simulink model "simulation_upgrade"  (R2024b)
settings: Solver=ode1be  StartTime=0.0  StopTime=10  FixedStep=0.001  RelTol=1e-3
model workspace (MAT data in the model file):
  AMP = 1
  FREQ = 1
  i_abc = 1
values from neighbouring files (symbols this model uses):
  v_WLTP = [0 0 0 0 0 0 0 0 0 0 0 0 ... (180001 elements, 1x180001)]    [v_WLTP.mat]
undefined symbols (not defined in the file or in its folder): A, a_sig, b_sig, C1, C2, C3, Cd, CG_z, downshift, Drive_wheel, Driveshaft, f_blend, f_OVD, fo, front_seat_dist, fs, g, Gearbox, i, i_sig, Inclination, Inertia, Jr2, K, m, M_curve_1, M_curve_2, m_driver, M_N_1, M_N_2, mi_c, mi_s, Mode, N_clutch, n_curve_1, n_curve_2, n_driver, n_max_1, n_max_2, n_shift, n_surfaces, Pl, Planetary, r_eq_clutch, r_geom, r_wheel, rho, Shaft, shift_time, sigma0, sigma1, sigma2, slope_angle, Stage1, Stage2, Stage3, upshift, v0, vel_wind, vs ... (+5)
libraries: simulink x29, slpidlib x3
(part 6 of 9)

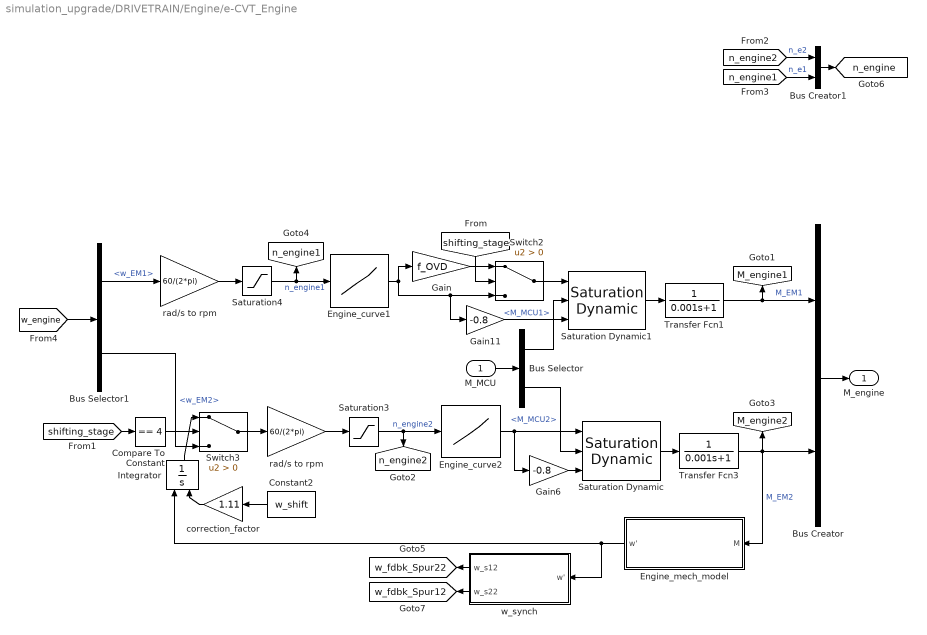
== system simulation_upgrade/DRIVETRAIN/Engine/e-CVT_Engine ==
  M_MCU : Inport
  Bus Creator : BusCreator  Inputs=2
  Bus Creator1 : BusCreator  Inputs=2
  Bus Selector : BusSelector  OutputSignals=M_MCU1,M_MCU2
  Bus Selector1 : BusSelector  OutputSignals=w_EM1,w_EM2
  Compare To Constant : simulink/Logic and Bit Operations/Compare To Constant  relop===  const=4  OutDataTypeStr=boolean
  Constant2 : Constant  Value=w_shift
  Engine_curve1 : Lookup_n-D  NumberOfTableDimensions=1  BreakpointsForDimension1=n_curve_1  Table=M_curve_1  InternalRulePriority=Speed  RndMeth=Simplest
  Engine_curve2 : Lookup_n-D  NumberOfTableDimensions=1  BreakpointsForDimension1=n_curve_2  Table=M_curve_2  InternalRulePriority=Speed  RndMeth=Simplest
  Engine_mech_model : Subsystem  mask{J_S1=Stage1.Spur1.J, J_S2=Stage1.Spur2.J, J_S11=Stage2.Spur11.J, J_S21=Stage2.Spur21.J, J_S12=Stage2.Spur12.J, J_S22=Stage2.Spur22.J, Jshaft=Shaft.J}
      mask prompts: J_S1 "Stage 1 Spur 1 Inertia"; J_S2 "Stage 1 Spur 2 Inertia"; J_S11 "Stage 2 Spur 11 Inertia"; J_S21 "Stage 2 Spur 21 Inertia"; J_S12 "Stage 2 Spur 12 Inertia"; J_S22 "Stage 2 Spur 22 Inertia"; Jshaft "Shaft Inertia"
  Gain : Gain  Gain=f_OVD
  Gain11 : Gain  Gain=-0.8
  Gain6 : Gain  Gain=-0.8
  Integrator : Integrator  InitialConditionSource=external
  Saturation Dynamic : simulink/Discontinuities/Saturation Dynamic  OutMin=[]  OutMax=[]  OutDataTypeStr=Inherit: Same as second input  OutDataType=fixdt(1, 16)  OutScaling=2^-10  DoSatur=off
  Saturation Dynamic1 : simulink/Discontinuities/Saturation Dynamic  OutMin=[]  OutMax=[]  OutDataTypeStr=Inherit: Same as second input  OutDataType=fixdt(1, 16)  OutScaling=2^-10  DoSatur=off
  Saturation3 : Saturate  UpperLimit=n_max_2
  Saturation4 : Saturate  UpperLimit=n_max_2
  Switch2 : Switch  Criteria=u2 > Threshold  SaturateOnIntegerOverflow=off  InputSameDT=off
  Switch3 : Switch  Criteria=u2 > Threshold  SaturateOnIntegerOverflow=off  InputSameDT=off
  Transfer Fcn1 : TransferFcn  Denominator=[0.001 1]
  Transfer Fcn3 : TransferFcn  Denominator=[0.001 1]
  "correction_factor " : Gain  Gain=1.11
  rad/s to rpm : Gain  Gain=60/(2*pi)
  "rad/s to rpm " : Gain  Gain=60/(2*pi)
  w_synch : Subsystem
      settings: PortSchema="{\"entries\":[{\"content\":{\"sides\":[{\"content\":{\"connectorIds\":[\"Out1\",\"Out2\"]},\"type\":\"ConnectorPlacement.EquallySpacedRectSide\",\"uuid\":\"0c74f9d6-4dd7-46ca-984a-3872ca362183\"},{\"content\":{\"connectorIds\":[\"In1\"],\"side\":\"RIGHT\"},\"type\":\"ConnectorPlacement.EquallySpacedRectSide\",\"uuid\":\"545eaab0-161e-407a-bd7a-8511cf00bcf5\"},{\"content\":{\"side\":\"TOP\"},\"type\":\"ConnectorPlacement.EquallySpacedRectSide\",\"uuid\":\"a44ef98a-c6fa-4a8f-9ec6-3c467f201227\"}]},\"type\":\"ConnectorPlacement.EquallySpacedConnector\",\"uuid\":\"6cdff010-dc2a-4ca6-852d-068deaf42780\"}],\"packageUris\":[\"http://schema.mathworks.com/mf0/Connector/R2020b\"],\"version\":\"1.0\"}"
      mask Display: image('branco.png');
  M_engine : Outport
  tag scope: M_engine1=global, M_engine2=global, n_engine1=global, n_engine2=global, n_engine=global, w_fdbk_Spur12=global, w_fdbk_Spur22=global
  wires:
  w_synch/2(w_s22) -> [w_fdbk_Spur12]
  w_synch/1(w_s12) -> [w_fdbk_Spur22]
  Gain11/1 -> Saturation Dynamic1/3
  rad/s to rpm/1 -> Saturation4/1
  Saturation4/1 -> [n_engine1], Engine_curve1/1  "n_engine1"
  Saturation Dynamic1/1 -> Transfer Fcn1/1
  "correction_factor "/1 -> Integrator/2
  Constant2/1 -> "correction_factor "/1
  Bus Selector1/2 -> Switch3/3  "<w_EM2>"
  Saturation Dynamic/1 -> Transfer Fcn3/1
  Gain6/1 -> Saturation Dynamic/3
  Bus Creator1/1 -> [n_engine]
  [n_engine1] -> Bus Creator1/2  "n_e1"
  [n_engine2] -> Bus Creator1/1  "n_e2"
  Integrator/1 -> Switch3/1
  Transfer Fcn3/1 -> [M_engine2], Engine_mech_model/1(M), Bus Creator/2  "M_EM2"
  Engine_mech_model/1(w') -> Integrator/1, w_synch/1(w')
  [shifting_stage] -> Compare To Constant/1
  Compare To Constant/1 -> Switch3/2
  Switch3/1 -> "rad/s to rpm "/1
  [shifting_stage] -> Switch2/2
  Gain/1 -> Switch2/1
  Switch2/1 -> Saturation Dynamic1/1
  Bus Creator/1 -> M_engine/1
  [w_engine] -> Bus Selector1/1
  Bus Selector/2 -> Saturation Dynamic/2  "<M_MCU2>"
  Saturation3/1 -> [n_engine2], Engine_curve2/1  "n_engine2"
  Engine_curve2/1 -> Saturation Dynamic/1, Gain6/1
  "rad/s to rpm "/1 -> Saturation3/1
  Bus Selector1/1 -> rad/s to rpm/1  "<w_EM1>"
  M_MCU/1 -> Bus Selector/1
  Bus Selector/1 -> Saturation Dynamic1/2  "<M_MCU1>"
  Engine_curve1/1 -> Gain/1, Gain11/1, Switch2/3
  Transfer Fcn1/1 -> [M_engine1], Bus Creator/1  "M_EM1"

== system simulation_upgrade/DRIVETRAIN/Transmission/Differential and Driveshafts ==
  M_Diff : Inport
  Bus Creator : BusCreator  Inputs=4
  Gain2 : Gain  Gain=0.5
  Gain3 : Gain  Gain=0.5
  Gain4 : Gain  Gain=0.5
  Sum : Sum  Inputs=+|+
  Torsional_stiffness_left_output_shaft : Subsystem  mask{c=Driveshaft.Right.c, d=Driveshaft.Right.d, J=Driveshaft.Right.J}
      mask prompts: c "Shaft_Stiffness_Nm/rad"; d "Shaft_Damping_Nms/rad"; J "Inertia_kgm^2"
      settings: PortSchema="{\"entries\":[{\"content\":{\"sides\":[{\"content\":{\"connectorIds\":[\"In1\",\"Out2\"]},\"type\":\"ConnectorPlacement.EquallySpacedRectSide\",\"uuid\":\"898fedf9-82f7-4bc2-bf05-880de36b191d\"},{\"content\":{\"connectorIds\":[\"Out1\",\"In2\"],\"side\":\"RIGHT\"},\"type\":\"ConnectorPlacement.EquallySpacedRectSide\",\"uuid\":\"50317b6c-245f-4bd1-a8cd-7a774957ae86\"},{\"content\":{\"side\":\"TOP\"},\"type\":\"ConnectorPlacement.EquallySpacedRectSide\",\"uuid\":\"ff1de2a1-7305-40d8-9e1f-fd0fa1e7d830\"}]},\"type\":\"ConnectorPlacement.EquallySpacedConnector\",\"uuid\":\"6ce82d73-f3da-4f59-9039-464a6ef3e9c5\"}],\"packageUris\":[\"http://schema.mathworks.com/mf0/Connector/R2020b\"],\"version\":\"1.0\"}"
      mask Display: image('images/torsion.png');
  Torsional_stiffness_right_output_shaft : Subsystem  mask{c=Driveshaft.Right.c, d=Driveshaft.Right.d, J=Driveshaft.Right.J}
      mask prompts: c "Shaft_Stiffness_Nm/rad"; d "Shaft_Damping_Nms/rad"; J "Inertia_kgm^2"
      settings: PortSchema="{\"entries\":[{\"content\":{\"sides\":[{\"content\":{\"connectorIds\":[\"In1\",\"Out2\"]},\"type\":\"ConnectorPlacement.EquallySpacedRectSide\",\"uuid\":\"898fedf9-82f7-4bc2-bf05-880de36b191d\"},{\"content\":{\"connectorIds\":[\"Out1\",\"In2\"],\"side\":\"RIGHT\"},\"type\":\"ConnectorPlacement.EquallySpacedRectSide\",\"uuid\":\"50317b6c-245f-4bd1-a8cd-7a774957ae86\"},{\"content\":{\"side\":\"TOP\"},\"type\":\"ConnectorPlacement.EquallySpacedRectSide\",\"uuid\":\"ff1de2a1-7305-40d8-9e1f-fd0fa1e7d830\"}]},\"type\":\"ConnectorPlacement.EquallySpacedConnector\",\"uuid\":\"6ce82d73-f3da-4f59-9039-464a6ef3e9c5\"}],\"packageUris\":[\"http://schema.mathworks.com/mf0/Connector/R2020b\"],\"version\":\"1.0\"}"
      mask Display: image('images/torsion.png');
  eff : Gain  Gain=0.98
  "eff " : Gain  Gain=0.98
  M_tra : Outport
  tag scope: M_diff=global, M_tra=global, w_fdbk_axleL=global, w_fdbk_axleR=global, w_fdbk_diff=global
  wires:
  "eff "/1 -> Bus Creator/4  "M_axleR"
  eff/1 -> Bus Creator/1  "M_axleL"
  Bus Creator/1 -> M_tra/1, [M_tra]
  [M_diff] -> Bus Creator/3
  [M_GB] -> Bus Creator/2
  [w_fdbk_tire] -> Torsional_stiffness_left_output_shaft/2(Speed_fdbk), Torsional_stiffness_right_output_shaft/2(Speed_fdbk)
  Torsional_stiffness_right_output_shaft/1(Torque_out) -> "eff "/1
  Torsional_stiffness_left_output_shaft/1(Torque_out) -> eff/1
  Sum/1 -> Gain3/1
  Gain4/1 -> Torsional_stiffness_right_output_shaft/1(Torque_in)  "M_axleR"
  Torsional_stiffness_left_output_shaft/2(phi_shaft_R_dot) -> Sum/1, [w_fdbk_axleL]
  Gain3/1 -> [w_fdbk_diff]
  M_Diff/1 -> Gain4/1, Gain2/1, [M_diff]  "M_diff"
  Torsional_stiffness_right_output_shaft/2(phi_shaft_R_dot) -> [w_fdbk_axleR], Sum/2
  Gain2/1 -> Torsional_stiffness_left_output_shaft/1(Torque_in)  "M_axleL"

== system simulation_upgrade/DRIVETRAIN/Transmission/Gearbox ==
  note: 1) Add Subsystem or Model blocks as valid variant choices.
      | 2) You cannot connect blocks at this level. At simulation, connectivity is automatically
      | determined, based on the active variant and port name matching.
  M_engine : Inport
  AMT : Subsystem  VariantControl=Gearbox == 2
      mask Display: image('images/clutch.jpg');
  AT : Subsystem  VariantControl=Gearbox == 1
      mask Display: image('images/planetary.png');
  DCT : Subsystem  VariantControl=Gearbox == 3
      mask Display: image('images/dual_clutch.png');
  TDT : Subsystem  VariantControl=Gearbox == 4
      mask Display: image('images/dog_clutch.png');
  e-CVT : Subsystem  VariantControl=Gearbox == 5
      mask Display: image('images/e-CVT.png');
  M_Diff : Outport

== system simulation_upgrade/DRIVETRAIN/Wheel Model/Front Wheels ==
  Vload : Inport
  M_tra : Inport  Port=2
  M_break : Inport  Port=3
  Divide1 : Product  Inputs=/*
  Dynamic Radius : Subsystem
  Wheel Torque : Subsystem
  F_front_wheels : Outport
  wires:
  M_tra/1 -> Wheel Torque/1(M_tra)
  M_break/1 -> Wheel Torque/2(M_break)
  Wheel Torque/1(M_front_wheels) -> Divide1/2
  Vload/1 -> Dynamic Radius/1(V_load)
  Dynamic Radius/1(r_dynamic_front) -> Divide1/1
  Divide1/1 -> F_front_wheels/1

== system simulation_upgrade/DRIVETRAIN/Wheel Model/Rear Wheels ==
  M_tra : Inport
  M_break : Inport  Port=2
  Vload : Inport  Port=3
  Divide1 : Product  Inputs=/*
  Dynamic Radius : Subsystem
  Wheel Torque : Subsystem
  F_rear_wheels : Outport
  wires:
  Vload/1 -> Dynamic Radius/1(V_load)
  Divide1/1 -> F_rear_wheels/1
  Dynamic Radius/1(r_dynamic_rear) -> Divide1/1
  M_tra/1 -> Wheel Torque/1(M_tra)
  M_break/1 -> Wheel Torque/2(M_break)
  Wheel Torque/1(M_rear_wheels) -> Divide1/2

== system simulation_upgrade/DYNAMICS/Vehicle Dynamics/Effective mass ==
  " 2nd engine gearbox inertia" : Constant  Commented=on  Value=Inertia.Second_Engine_Gearbox
  Add : Sum
  Add1 : Sum  Commented=on  Inputs=+++
  Add2 : Sum  Commented=on
  Add3 : Sum  Commented=on  Inputs=+++
  Add4 : Sum  Commented=on
  Add5 : Sum  Commented=on
  Constant : Constant  Value=m
  Constant1 : Constant  Commented=on  Value=r_wheel
  Divide : Product  Commented=on  Inputs=*/
  From : From  Commented=on  GotoTag=C2_ist  TagVisibility=global
  Manual Switch : ManualSwitch
  Multiport Switch : MultiPortSwitch  Commented=on  DataPortOrder=Zero-based contiguous  zeroidx=on  SaturateOnIntegerOverflow=off  InputSameDT=off
  Output shaft inertia : Constant  Commented=on  Value=Inertia.Output_Shaft
  Scope : Scope
  Square : Math  Commented=on  Operator=square
  Stage 1 - 1st Gear Inertia : Constant  Commented=on  Value=Inertia.Gearbox1.Stage_1_1st_Gear
  Stage 1 - 2nd Gear Inertia1 : Constant  Commented=on  Value=Inertia.Gearbox1.Stage_1_2nd_Gear
  Stage 2 - 1st Gear Inertia : Constant  Commented=on  Value=Inertia.Gearbox1.Stage_2_1st_Gear
  Stage 2 - 2nd Gear Inertia : Constant  Commented=on  Value=Inertia.Gearbox1_Stage_2_2nd_Gear
  Stage 3 : Constant  Commented=on  Value=Inertia.Gearbox1_Stage_3
  m_eff : Outport
  tag scope: m_eff=global
  wires:
  Add/1 -> Manual Switch/2
  Add4/1 -> Multiport Switch/3  "1st gear"
  Multiport Switch/1 -> Divide/1  "I_eff"
  Divide/1 -> Add/2
  Square/1 -> Divide/2
  Add5/1 -> Multiport Switch/4  "2nd gear"
  Output shaft inertia/1 -> Add2/1
  From/1 -> Multiport Switch/1
  Add2/1 -> Add5/1, Add4/1, Multiport Switch/2  "neutral"
  Constant/1 -> Manual Switch/1, Add/1
  Constant1/1 -> Square/1
  Add3/1 -> Add5/2  "2nd gear gearbox inertia"
  Add1/1 -> Add4/2  "1st gear gearbox inertia"
  " 2nd engine gearbox inertia"/1 -> Add2/2
  Stage 1 - 1st Gear Inertia/1 -> Add1/1
  Stage 3/1 -> Add1/3, Add3/1
  Stage 2 - 1st Gear Inertia/1 -> Add1/2
  Stage 2 - 2nd Gear Inertia/1 -> Add3/3
  Stage 1 - 2nd Gear Inertia1/1 -> Add3/2
  Manual Switch/1 -> Scope/1, [m_eff], m_eff/1

== system simulation_upgrade/PANEL/Pretty shot/Aerodynamic Forces  ==
  " " : Inport
  "  " : Outport
  wires:
  " "/1 -> "  "/1

== system simulation_upgrade/PANEL/Pretty shot/Engine(s)  ==
  "  " : Inport
  "             " : Outport
  "              " : Outport  Port=2
  wires:
  "  "/1 -> "             "/1

== system simulation_upgrade/PANEL/Pretty shot/Inclination  ==
  Constant : Constant
  "   " : Outport
  " " : Outport  Port=2
  wires:
  Constant/1 -> " "/1, "   "/1

== system simulation_upgrade/PANEL/Pretty shot/Load Transfer  ==
  " " : Inport
  "      " : Inport  Port=2
  Terminator : Terminator
  "  " : Outport
  wires:
  "      "/1 -> Terminator/1
  " "/1 -> "  "/1

== system simulation_upgrade/PANEL/Pretty shot/Main Control Unit  ==
  " " : Inport
  "   " : Inport  Port=2
  Chart : Stateflow chart  Commented=on  TreatAsAtomicUnit=on
  "  " : Outport
  "    " : Outport  Port=2
  wires:
  Chart/1("  ") -> "  "/1
  Chart/2("    ") -> "    "/1
  "   "/1 -> Chart/2("   ")
  " "/1 -> Chart/1(" ")

== system simulation_upgrade/PANEL/Pretty shot/Speed Profile  ==
  Constant : Constant
  " " : Outport
  wires:
  Constant/1 -> " "/1

== system simulation_upgrade/PANEL/Pretty shot/Speed control  ==
  "    " : Inport
  " " : Inport  Port=2
  "         " : Outport
  "        " : Outport  Port=2
  wires:
  " "/1 -> "         "/1
  "    "/1 -> "        "/1

== system simulation_upgrade/PANEL/Pretty shot/Transmission  ==
  " " : Inport
  "     " : Inport  Port=2
  "    " : Inport  Port=3
  "   " : Inport  Port=4
  Variant Subsystem : Subsystem  Commented=on  Variant=on
  "  " : Outport
  wires:
  " "/1 -> "  "/1

== system simulation_upgrade/PANEL/Pretty shot/Vehicle Dynamics  ==
  " " : Inport
  "  " : Outport
  wires:
  " "/1 -> "  "/1

== system simulation_upgrade/PANEL/Pretty shot/Wheel Model  ==
  "  " : Inport
  " " : Inport  Port=2
  "   " : Outport
  "    " : Outport  Port=2
  wires:
  "  "/1 -> "    "/1
  " "/1 -> "   "/1

== system simulation_upgrade/CONTROLS/Main Control Unit/AMT_MCU/Subsystem ==
  clutchSet : Inport
  Clock : Clock
  Delay : Delay  DelayLength=1  InitialCondition=1  InputProcessing=Columns as channels (frame based)
  Equal1 : RelationalOperator  Operator=<=  OutDataTypeStr=boolean  RndMeth=Simplest  InputSameDT=off
  Equal2 : RelationalOperator  OutDataTypeStr=boolean  RndMeth=Simplest  InputSameDT=off
  Manual Switch1 : ManualSwitch
  Polynomial : Subsystem
  Product : Product
  Scope : Scope  NumInputPorts=3
  Scope2 : Scope
  Scope3 : Scope
  Sigmoid : Subsystem
  Sum : Sum  Inputs=|-+
  Sum2 : Sum  Inputs=++|
  Switch : Switch  Criteria=u2 > Threshold  SaturateOnIntegerOverflow=off  InputSameDT=off
  Switch1 : Switch  Threshold=1  SaturateOnIntegerOverflow=off  InputSameDT=off
  Transport Delay : TransportDelay  DelayTime=0.001  InitialOutput=1
  signal_register : Subsystem
  time_register : Subsystem
  C2 : Outport
  wires:
  Sum/1 -> Sigmoid/1(" "), Polynomial/1(" ")
  Switch1/1 -> Transport Delay/1
  Product/1 -> Sum2/2
  time_register/1(t0) -> Scope2/1, Sum/1
  Equal2/1 -> Switch/3
  Clock/1 -> time_register/1(t), Sum/2
  Delay/1 -> Scope3/1, time_register/Trigger, signal_register/1(signal), signal_register/Trigger, Scope/3, Switch1/1, Equal2/1, Equal1/1
  clutchSet/1 -> Delay/1
  Polynomial/1("  ") -> Manual Switch1/1
  signal_register/1(previous_value) -> Sum2/1
  Sigmoid/1("  ") -> Manual Switch1/2
  Transport Delay/1 -> Scope/2, C2/1
  Equal1/1 -> Switch/1
  Sum2/1 -> Equal1/2, Equal2/2, Scope/1, Switch1/3
  signal_register/2(difference) -> Switch/2, Product/1
  Manual Switch1/1 -> Product/2
  Switch/1 -> Switch1/2

== system simulation_upgrade/CONTROLS/Main Control Unit/AT_MCU/Clutch_Profile ==
  clutch2set : Inport
  clutch1set : Inport  Port=2
  Manual Switch : ManualSwitch  CurrentSetting=0
  Manual Switch1 : ManualSwitch  CurrentSetting=0
  polynomial_s_response : Subsystem
  polynomial_s_response1 : Subsystem
  sigmoid_response : Subsystem
  sigmoid_response1 : Subsystem
  Out1 : Outport
  Out2 : Outport  Port=2
  wires:
  polynomial_s_response/1(Out1) -> Manual Switch/2
  sigmoid_response/1(Out1) -> Manual Switch/1
  clutch2set/1 -> polynomial_s_response1/1(clutch2set), sigmoid_response1/1(clutch2set)
  polynomial_s_response1/1(Out1) -> Manual Switch1/2
  sigmoid_response1/1(Out1) -> Manual Switch1/1
  clutch1set/1 -> sigmoid_response/1(clutch1set), polynomial_s_response/1(clutch1set)
  Manual Switch1/1 -> Out1/1  "c2"
  Manual Switch/1 -> Out2/1  "c1"

== system simulation_upgrade/CONTROLS/Main Control Unit/AT_MCU/Shifting Impulses ==
  n_engine : Inport
  shiftng_stage : Inport  Port=2
  C2 : Inport  Port=3
  AND : Logic  Inputs=3  IconShape=distinctive  AllPortsSameDT=off  OutDataTypeStr=boolean
  AND1 : Logic  Inputs=4  IconShape=distinctive  AllPortsSameDT=off  OutDataTypeStr=boolean
  Compare To Constant : simulink/Logic and Bit Operations/Compare To Constant  relop===  const=0  OutDataTypeStr=boolean
  Compare To Constant1 : simulink/Logic and Bit Operations/Compare To Constant  relop=<  const=2000  OutDataTypeStr=boolean
  Compare To Constant2 : simulink/Logic and Bit Operations/Compare To Constant  relop=>=  const=n_shift  OutDataTypeStr=boolean
  Compare To Constant3 : simulink/Logic and Bit Operations/Compare To Constant  relop===  const=2  OutDataTypeStr=boolean
  Compare To Constant4 : simulink/Logic and Bit Operations/Compare To Constant  relop===  const=1  OutDataTypeStr=boolean
  Compare To Constant5 : simulink/Logic and Bit Operations/Compare To Constant  relop=<  const=0  OutDataTypeStr=boolean
  Delay : Delay  DelayLength=1
  Delay2 : Delay  DelayLength=1
  Manual Switch : ManualSwitch  CurrentSetting=0
  Manual Switch1 : ManualSwitch
  Scope : Scope
  Scope2 : Scope
  Zero1 : Constant  Value=0  OutDataTypeStr=Inherit: Inherit via back propagation
  downshift impulse : Subsystem
  upshift impulse : Subsystem
  upshift command : Outport
  downshift command : Outport  Port=2
  wires:
  C2/1 -> Compare To Constant3/1, Compare To Constant4/1
  Compare To Constant3/1 -> AND1/2
  AND1/1 -> downshift impulse/1(Event)
  Compare To Constant2/1 -> AND/2
  upshift impulse/1(Impulse) -> Delay2/1, Scope/1
  Compare To Constant/1 -> AND/3, AND1/1
  AND/1 -> upshift impulse/1(Event)
  downshift impulse/1(Impulse) -> Delay/1, Scope2/1
  Delay/1 -> Manual Switch/2
  Compare To Constant1/1 -> AND1/3
  Manual Switch/1 -> downshift command/1
  shiftng_stage/1 -> Compare To Constant/1
  [acc] -> Compare To Constant5/1
  n_engine/1 -> Compare To Constant1/1, Compare To Constant2/1
  Compare To Constant5/1 -> AND1/4
  Delay2/1 -> Manual Switch1/1
  Manual Switch1/1 -> upshift command/1
  Zero1/1 -> Manual Switch/1, Manual Switch1/2
  Compare To Constant4/1 -> AND/1

== system simulation_upgrade/CONTROLS/Main Control Unit/CVT_MCU/Torque Split ==
  M_Set_SC : Inport
  M_EM2 : Inport  Port=2
  GreaterThan : RelationalOperator  Operator=>  OutDataTypeStr=boolean  RndMeth=Simplest  InputSameDT=off
  M_N_2 : Step  Time=0  After=M_N_2  SampleTime=0
  Recuperation Limit : Saturate  UpperLimit=0  LowerLimit=-80
  Recuperation Limit1 : Saturate  UpperLimit=0  LowerLimit=-80
  Saturation : Saturate  UpperLimit=M_N_1  LowerLimit=0
  Saturation1 : Saturate  UpperLimit=M_N_2  LowerLimit=0
  Subtract : Sum  Inputs=+-
  Subtract1 : Sum  Inputs=-+
  Switch : Switch  Criteria=u2 > Threshold  SaturateOnIntegerOverflow=off  InputSameDT=off
  Switch2 : Switch  Criteria=u2 > Threshold  SaturateOnIntegerOverflow=off  InputSameDT=off
  M_Set_1 : Outport
  M_Set_2 : Outport  Port=2
  wires:
  Recuperation Limit1/1 -> Switch/3
  Saturation1/1 -> Switch2/1
  Subtract/1 -> Recuperation Limit1/1
  M_EM2/1 -> Subtract1/1
  Switch/1 -> M_Set_1/1
  Saturation/1 -> Switch/1
  Recuperation Limit/1 -> Subtract/2, Switch2/3
  Switch2/1 -> M_Set_2/1
  GreaterThan/1 -> Switch/2
  Subtract1/1 -> Saturation/1
  M_Set_SC/1 -> Recuperation Limit/1, Saturation1/1, Switch2/2, Subtract/1, Subtract1/2, GreaterThan/1
  M_N_2/1 -> GreaterThan/2

== system simulation_upgrade/CONTROLS/Main Control Unit/DCT_MCU/Subsystem ==
  clutchSet : Inport
  Clock : Clock
  Delay : Delay  DelayLength=1  InitialCondition=1  InputProcessing=Columns as channels (frame based)
  Equal1 : RelationalOperator  Operator=<=  OutDataTypeStr=boolean  RndMeth=Simplest  InputSameDT=off
  Equal2 : RelationalOperator  OutDataTypeStr=boolean  RndMeth=Simplest  InputSameDT=off
  Hyperbolic : Subsystem
  Manual Switch1 : ManualSwitch  CurrentSetting=0
  Polynomial : Subsystem
  Product : Product
  Scope : Scope  NumInputPorts=3
  Scope2 : Scope
  Scope3 : Scope
  Sigmoid : Subsystem
  Sum : Sum  Inputs=|-+
  Sum2 : Sum  Inputs=++|
  Switch : Switch  Criteria=u2 > Threshold  SaturateOnIntegerOverflow=off  InputSameDT=off
  Switch1 : Switch  Threshold=1  SaturateOnIntegerOverflow=off  InputSameDT=off
  Transport Delay : TransportDelay  DelayTime=0.001  InitialOutput=1
  signal_register : Subsystem
  time_register : Subsystem
  C2 : Outport
  wires:
  Sum/1 -> Hyperbolic/1(" "), Polynomial/1(" ")
  Switch1/1 -> Transport Delay/1
  Product/1 -> Sum2/2
  time_register/1(t0) -> Scope2/1, Sum/1
  Equal2/1 -> Switch/3
  Clock/1 -> time_register/1(t), Sum/2
  Polynomial/1("  ") -> Manual Switch1/1
  signal_register/1(previous_value) -> Sum2/1
  Sigmoid/1("  ") -> ?
  Transport Delay/1 -> Scope/2, C2/1
  Equal1/1 -> Switch/1
  Sum2/1 -> Equal1/2, Equal2/2, Scope/1, Switch1/3
  signal_register/2(difference) -> Switch/2, Product/1
  Manual Switch1/1 -> Product/2
  Switch/1 -> Switch1/2
  Hyperbolic/1("  ") -> Manual Switch1/2
  clutchSet/1 -> Delay/1
  Delay/1 -> time_register/Trigger, Scope/3, Switch1/1, Equal2/1, Equal1/1, signal_register/Trigger, signal_register/1(signal), Scope3/1

== system simulation_upgrade/CONTROLS/Main Control Unit/DCT_MCU/Subsystem1 ==
  clutchSet : Inport
  Clock : Clock
  Equal1 : RelationalOperator  Operator=<=  OutDataTypeStr=boolean  RndMeth=Simplest  InputSameDT=off
  Equal2 : RelationalOperator  OutDataTypeStr=boolean  RndMeth=Simplest  InputSameDT=off
  Hyperbolic : Subsystem
  Manual Switch1 : ManualSwitch
  Polynomial : Subsystem
  Product : Product
  Scope : Scope  NumInputPorts=3
  Scope2 : Scope
  Scope3 : Scope
  Sigmoid : Subsystem
  Sum : Sum  Inputs=|-+
  Sum2 : Sum  Inputs=++|
  Switch : Switch  Criteria=u2 > Threshold  SaturateOnIntegerOverflow=off  InputSameDT=off
  Switch1 : Switch  Threshold=1  SaturateOnIntegerOverflow=off  InputSameDT=off
  Transport Delay : TransportDelay  DelayTime=0.001
  signal_register : Subsystem
  time_register : Subsystem
  C2 : Outport
  wires:
  Switch/1 -> Switch1/2
  Manual Switch1/1 -> Product/2
  signal_register/2(difference) -> Product/1, Switch/2
  Sum2/1 -> Switch1/3, Scope/1, Equal2/2, Equal1/2
  Equal1/1 -> Switch/1
  Transport Delay/1 -> C2/1, Scope/2
  Sigmoid/1("  ") -> ?
  signal_register/1(previous_value) -> Sum2/1
  Polynomial/1("  ") -> Manual Switch1/1
  clutchSet/1 -> Equal1/1, Equal2/1, Switch1/1, Scope/3, signal_register/Trigger, signal_register/1(signal), time_register/Trigger, Scope3/1
  Clock/1 -> Sum/2, time_register/1(t)
  Equal2/1 -> Switch/3
  time_register/1(t0) -> Sum/1, Scope2/1
  Product/1 -> Sum2/2
  Switch1/1 -> Transport Delay/1
  Sum/1 -> Hyperbolic/1(" "), Polynomial/1(" ")
  Hyperbolic/1("  ") -> Manual Switch1/2

== system simulation_upgrade/CONTROLS/Main Control Unit/TDT_MCU/Torque Split ==
  M_Set_SC : Inport
  M_EM2 : Inport  Port=2
  GreaterThan : RelationalOperator  Operator=>  OutDataTypeStr=boolean  RndMeth=Simplest  InputSameDT=off
  M_N_2 : Step  Time=0  After=M_N_2  SampleTime=0
  Recuperation Limit : Saturate  UpperLimit=0  LowerLimit=-300
  Recuperation Limit1 : Saturate  UpperLimit=0  LowerLimit=-300
  Saturation : Saturate  UpperLimit=M_N_1  LowerLimit=0
  Saturation1 : Saturate  UpperLimit=M_N_2  LowerLimit=0
  Subtract : Sum  Inputs=+-
  Subtract1 : Sum  Inputs=-+
  Switch : Switch  Criteria=u2 > Threshold  SaturateOnIntegerOverflow=off  InputSameDT=off
  Switch2 : Switch  Criteria=u2 > Threshold  SaturateOnIntegerOverflow=off  InputSameDT=off
  M_Set_1 : Outport
  M_Set_2 : Outport  Port=2
  wires:
  Recuperation Limit1/1 -> Switch/3
  Saturation1/1 -> Switch2/1
  Subtract/1 -> Recuperation Limit1/1
  M_EM2/1 -> Subtract1/1
  Switch/1 -> M_Set_1/1
  Saturation/1 -> Switch/1
  Recuperation Limit/1 -> Subtract/2, Switch2/3
  Switch2/1 -> M_Set_2/1
  GreaterThan/1 -> Switch/2
  Subtract1/1 -> Saturation/1
  M_Set_SC/1 -> Recuperation Limit/1, Saturation1/1, Switch2/2, Subtract/1, Subtract1/2, GreaterThan/1
  M_N_2/1 -> GreaterThan/2

== system simulation_upgrade/DRIVETRAIN/Engine/AMT_Engine/Engine_mech_model ==
  M : Inport
  Constant : Constant  Value=Jr2+J_S1+Jshaft
  Constant2 : Constant  Value=J_S2+Jshaft+J_S11+J_S21
  Constant4 : Constant  Value=J_S22
  Constant5 : Constant  Value=J_S12
  Divide : Product  Inputs=*/
  Gain7 : Gain  Gain=1/i.S1^2
  Gain8 : Gain  Gain=1/i.S21^2
  Gain9 : Gain  Gain=1/i.S22^2
  Sum1 : Sum  Inputs=+|+
  Sum2 : Sum  Inputs=+|+
  Sum3 : Sum  Inputs=+|+
  w' : Outport
  wires:
  M/1 -> Divide/1
  Divide/1 -> w'/1
  Gain8/1 -> Sum1/2
  Gain9/1 -> Sum1/1
  Constant/1 -> Sum3/2
  Constant2/1 -> Gain7/1
  Constant4/1 -> Gain9/1
  Gain7/1 -> Sum3/1
  Sum1/1 -> Sum2/1
  Constant5/1 -> Gain8/1
  Sum3/1 -> Divide/2

== system simulation_upgrade/DRIVETRAIN/Engine/DCT_Engine/Engine_mech_model ==
  M : Inport
  Constant : Constant  Value=Jr2+J_S1+Jshaft
  Constant2 : Constant  Value=J_S2+Jshaft+J_S11+J_S21
  Constant4 : Constant  Value=J_S22
  Constant5 : Constant  Value=J_S12
  Divide : Product  Inputs=*/
  Gain7 : Gain  Gain=1/i.S1^2
  Gain8 : Gain  Gain=1/i.S21^2
  Gain9 : Gain  Gain=1/i.S22^2
  Sum1 : Sum  Inputs=+|+
  Sum2 : Sum  Inputs=+|+
  Sum3 : Sum  Inputs=+|+
  w' : Outport
  wires:
  Sum3/1 -> Divide/2
  Constant5/1 -> Gain8/1
  Sum1/1 -> Sum2/1
  Gain7/1 -> Sum3/1
  Constant4/1 -> Gain9/1
  Sum2/1 -> Gain7/1
  Constant2/1 -> Sum2/2
  Constant/1 -> Sum3/2
  Gain9/1 -> Sum1/1
  Gain8/1 -> Sum1/2
  Divide/1 -> w'/1
  M/1 -> Divide/1

== system simulation_upgrade/DRIVETRAIN/Engine/TDT_Engine/Engine_mech_model ==
  M : Inport
  Constant : Constant  Value=Jr2+J_S1+Jshaft
  Constant2 : Constant  Value=J_S2+Jshaft+J_S11+J_S21
  Constant4 : Constant  Value=J_S22
  Constant5 : Constant  Value=J_S12
  Divide : Product  Inputs=*/
  Gain7 : Gain  Gain=1/i.S1^2
  Gain8 : Gain  Gain=1/i.S21^2
  Gain9 : Gain  Gain=1/i.S22^2
  Sum1 : Sum  Inputs=+|+
  Sum2 : Sum  Inputs=+|+
  Sum3 : Sum  Inputs=+|+
  w' : Outport
  wires:
  M/1 -> Divide/1
  Divide/1 -> w'/1
  Gain8/1 -> Sum1/2
  Gain9/1 -> Sum1/1
  Constant/1 -> Sum3/2
  Constant2/1 -> Sum2/2
  Sum2/1 -> Gain7/1
  Constant4/1 -> Gain9/1
  Gain7/1 -> Sum3/1
  Sum1/1 -> Sum2/1
  Constant5/1 -> Gain8/1
  Sum3/1 -> Divide/2

== system simulation_upgrade/DRIVETRAIN/Engine/TDT_Engine/w_synch ==
  signal : Inport
  w' : Inport  Port=2
  Gain2 : Gain  Gain=1/i.S22
  Gain3 : Gain  Gain=i.S21*i.S1
  Gain5 : Gain  Gain=i.S22*i.S1
  Gain7 : Gain  Gain=1/i.S21
  Integrator1 : Integrator  ExternalReset=either  InitialConditionSource=external
  Integrator2 : Integrator  ExternalReset=either  InitialConditionSource=external
  Scope : Scope  NumInputPorts=2
  Scope1 : Scope  NumInputPorts=4
  Switch4 : Switch  Criteria=u2 > Threshold  SaturateOnIntegerOverflow=off  InputSameDT=off
  Switch5 : Switch  Criteria=u2 > Threshold  SaturateOnIntegerOverflow=off  InputSameDT=off
  Switch6 : Switch  Criteria=u2 > Threshold  SaturateOnIntegerOverflow=off  InputSameDT=off
  w_s22 : Outport
  w_s21 : Outport  Port=2
  wires:
  Switch5/1 -> Scope/2, w_s21/1
  Integrator1/1 -> Scope1/2, Switch4/1
  Gain3/1 -> Integrator2/1
  Switch4/1 -> w_s22/1, Scope/1
  signal/1 -> Switch4/2, Switch5/2, Switch6/3, Switch6/2, Integrator2/2, Integrator1/2
  Gain5/1 -> Integrator1/1
  [w_fdbk_GB2] -> Gain2/1, Gain7/1
  Gain2/1 -> Integrator1/3, Scope1/1, Switch4/3
  Gain7/1 -> Integrator2/3, Scope1/3, Switch5/3
  Integrator2/1 -> Scope1/4, Switch5/1
  w'/1 -> Switch6/1
  Switch6/1 -> Gain3/1, Gain5/1

== system simulation_upgrade/DRIVETRAIN/Engine/e-CVT_Engine/Engine_mech_model ==
  M : Inport
  Constant : Constant  Value=Jr2+J_S1+Jshaft
  Constant2 : Constant  Value=J_S2+Jshaft+J_S11+J_S21
  Constant4 : Constant  Value=J_S22
  Constant5 : Constant  Value=J_S12
  Divide : Product  Inputs=*/
  Gain7 : Gain  Gain=1/i.S1^2
  Gain8 : Gain  Gain=1/i.S21^2
  Gain9 : Gain  Gain=1/i.S22^2
  Sum1 : Sum  Inputs=+|+
  Sum2 : Sum  Inputs=+|+
  Sum3 : Sum  Inputs=+|+
  w' : Outport
  wires:
  Sum3/1 -> Divide/2
  Constant5/1 -> Gain8/1
  Sum1/1 -> Sum2/1
  Gain7/1 -> Sum3/1
  Constant4/1 -> Gain9/1
  Sum2/1 -> Gain7/1
  Constant2/1 -> Sum2/2
  Constant/1 -> Sum3/2
  Gain9/1 -> Sum1/1
  Gain8/1 -> Sum1/2
  Divide/1 -> w'/1
  M/1 -> Divide/1

== system simulation_upgrade/DRIVETRAIN/Engine/e-CVT_Engine/w_synch ==
  w' : Inport
  Compare To Constant1 : simulink/Logic and Bit Operations/Compare To Constant  relop===  const=4  OutDataTypeStr=boolean
  Constant : Constant  Value=w_shift
  Correction factor : Gain  Gain=1.11
  Gain1 : Gain  Gain=i.S1
  Gain10 : Gain  Gain=1/(i.S1*i.S21)
  Gain2 : Gain  Gain=1/i.S22
  Gain4 : Gain  Gain=i.S21
  Gain5 : Gain  Gain=i.S22
  Gain7 : Gain  Gain=1/i.S21
  Gain9 : Gain  Gain=1/(i.S1*i.S22)
  Integrator1 : Integrator  InitialConditionSource=external
  Integrator2 : Integrator  InitialConditionSource=external
  Switch4 : Switch  Criteria=u2 > Threshold  SaturateOnIntegerOverflow=off  InputSameDT=off
  Switch5 : Switch  Criteria=u2 > Threshold  SaturateOnIntegerOverflow=off  InputSameDT=off
  Switch6 : Switch  Criteria=u2 > Threshold  SaturateOnIntegerOverflow=off  InputSameDT=off
  w_s12 : Outport
  w_s22 : Outport  Port=2
  wires:
  Gain1/1 -> Gain5/1, Gain4/1
  Constant/1 -> Correction factor/1
  w'/1 -> Switch6/1
  Integrator2/1 -> Switch5/1
  Gain9/1 -> Integrator1/2
  Gain7/1 -> Switch5/3
  Switch6/1 -> Gain1/1
  Gain2/1 -> Switch4/3
  [w_fdbk_GB2] -> Gain2/1, Gain7/1
  [shifting_stage] -> Compare To Constant1/1
  Gain5/1 -> Integrator1/1
  Correction factor/1 -> Gain9/1, Gain10/1
  Compare To Constant1/1 -> Switch6/3, Switch6/2, Switch5/2, Switch4/2
  Switch4/1 -> w_s12/1
  Gain4/1 -> Integrator2/1
  Integrator1/1 -> Switch4/1
  Switch5/1 -> w_s22/1
  Gain10/1 -> Integrator2/2

== system simulation_upgrade/DRIVETRAIN/Transmission/Differential and Driveshafts/Torsional_stiffness_left_output_shaft ==
  Torque_in : Inport
  Speed_fdbk : Inport  Port=2
  Add2 : Sum  Inputs=+-
  Add4 : Sum  Inputs=+-
  Divide2 : Product  Inputs=*/
  Integrator5 : Integrator
  Integrator7 : Integrator
  Integrator8 : Integrator
  J1 : Constant  Value=J
  Scope1 : Scope  NumInputPorts=2
  Sum2 : Sum  Inputs=|+-
  Sum4 : Sum
  Transfer Fcn1 : TransferFcn  Denominator=[0.001 1]
  c_s : Gain  Gain=c
  d_s : Gain  Gain=d
  Torque_out : Outport
  phi_shaft_R_dot : Outport  Port=2
  wires:
  Transfer Fcn1/1 -> Integrator5/1
  Torque_in/1 -> Scope1/1, Sum2/1  "T_1"
  d_s/1 -> Sum4/1
  Sum4/1 -> Scope1/2, Sum2/2, Torque_out/1  "T_2"
  Integrator7/1 -> Add2/1  "phi_1"
  Divide2/1 -> Transfer Fcn1/1  "phi_1_dotdot"
  Speed_fdbk/1 -> Integrator8/1, Add4/2  "phi_2_dot"
  Add2/1 -> c_s/1
  Integrator8/1 -> Add2/2  "phi_2"
  c_s/1 -> Sum4/2
  Sum2/1 -> Divide2/1
  J1/1 -> Divide2/2
  Integrator5/1 -> Add4/1, Integrator7/1, phi_shaft_R_dot/1  "v_fdbk_axleR"
  Add4/1 -> d_s/1

== system simulation_upgrade/DRIVETRAIN/Transmission/Differential and Driveshafts/Torsional_stiffness_right_output_shaft ==
  Torque_in : Inport
  Speed_fdbk : Inport  Port=2
  Add2 : Sum  Inputs=+-
  Add4 : Sum  Inputs=+-
  Divide2 : Product  Inputs=*/
  Integrator5 : Integrator
  Integrator7 : Integrator
  Integrator8 : Integrator
  J1 : Constant  Value=J
  Sum2 : Sum  Inputs=|+-
  Sum4 : Sum
  Transfer Fcn1 : TransferFcn  Denominator=[0.001 1]
  c_s : Gain  Gain=c
  d_s : Gain  Gain=d
  Torque_out : Outport
  phi_shaft_R_dot : Outport  Port=2
  wires:
  Add4/1 -> d_s/1
  Integrator5/1 -> phi_shaft_R_dot/1, Integrator7/1, Add4/1  "v_fdbk_axleR"
  J1/1 -> Divide2/2
  Sum2/1 -> Divide2/1
  c_s/1 -> Sum4/2
  Integrator8/1 -> Add2/2  "phi_2"
  Add2/1 -> c_s/1
  Speed_fdbk/1 -> Add4/2, Integrator8/1  "phi_2_dot"
  Divide2/1 -> Transfer Fcn1/1  "a_axle"
  Integrator7/1 -> Add2/1  "phi_1"
  Sum4/1 -> Torque_out/1, Sum2/2
  d_s/1 -> Sum4/1
  Torque_in/1 -> Sum2/1
  Transfer Fcn1/1 -> Integrator5/1

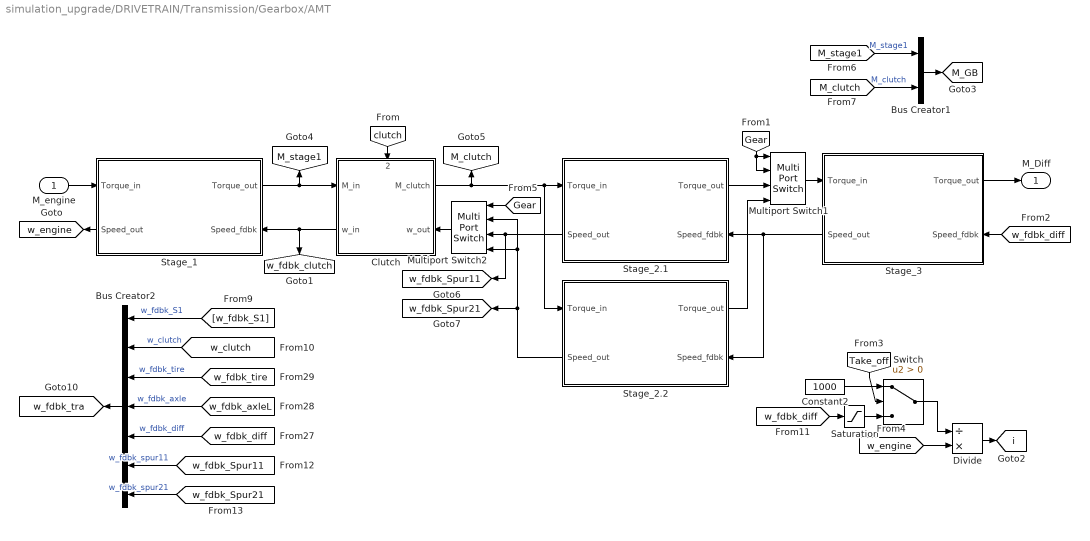
== system simulation_upgrade/DRIVETRAIN/Transmission/Gearbox/AMT ==
  M_engine : Inport
  Bus Creator1 : BusCreator  Inputs=2
  Bus Creator2 : BusCreator  Inputs=7
  Clutch : Subsystem
      settings: PortSchema="{\"entries\":[{\"content\":{\"sides\":[{\"content\":{\"connectorIds\":[\"In1\",\"Out2\"]},\"type\":\"ConnectorPlacement.EquallySpacedRectSide\",\"uuid\":\"d6060937-6a70-4d8f-85b8-f3c9c5d18f93\"},{\"content\":{\"connectorIds\":[\"Out1\",\"In3\"],\"side\":\"RIGHT\"},\"type\":\"ConnectorPlacement.EquallySpacedRectSide\",\"uuid\":\"5f6b068d-fc68-4249-8013-bc3df4965ca3\"},{\"content\":{\"connectorIds\":[\"In2\"],\"side\":\"TOP\"},\"type\":\"ConnectorPlacement.EquallySpacedRectSide\",\"uuid\":\"81b536de-881e-418d-8c02-7373631e1270\"}]},\"type\":\"ConnectorPlacement.EquallySpacedConnector\",\"uuid\":\"48438dfd-c2d0-4ff7-b57e-a1bd101206eb\"}],\"packageUris\":[\"http://schema.mathworks.com/mf0/Connector/R2020b\"],\"version\":\"1.0\"}"
      mask Display: image('images/clutch.jpg');
  Constant2 : Constant  Value=1000
  Divide : Product  Inputs=/*
  Multiport Switch1 : MultiPortSwitch  DataPortOrder=Zero-based contiguous  zeroidx=on  SaturateOnIntegerOverflow=off  InputSameDT=off
  Multiport Switch2 : MultiPortSwitch  DataPortOrder=Zero-based contiguous  zeroidx=on  SaturateOnIntegerOverflow=off  InputSameDT=off
  Saturation : Saturate  UpperLimit=1000000  LowerLimit=1
  Stage_1 : Subsystem  Variant=on
      settings: PortSchema="{\"entries\":[{\"content\":{\"sides\":[{\"content\":{\"connectorIds\":[\"In1\",\"Out2\"]},\"type\":\"ConnectorPlacement.EquallySpacedRectSide\",\"uuid\":\"898fedf9-82f7-4bc2-bf05-880de36b191d\"},{\"content\":{\"connectorIds\":[\"Out1\",\"In2\"],\"side\":\"RIGHT\"},\"type\":\"ConnectorPlacement.EquallySpacedRectSide\",\"uuid\":\"50317b6c-245f-4bd1-a8cd-7a774957ae86\"},{\"content\":{\"side\":\"TOP\"},\"type\":\"ConnectorPlacement.EquallySpacedRectSide\",\"uuid\":\"ff1de2a1-7305-40d8-9e1f-fd0fa1e7d830\"}]},\"type\":\"ConnectorPlacement.EquallySpacedConnector\",\"uuid\":\"6ce82d73-f3da-4f59-9039-464a6ef3e9c5\"}],\"packageUris\":[\"http://schema.mathworks.com/mf0/Connector/R2020b\"],\"version\":\"1.0\"}"
      mask Display: image('images/branco.png');
  Stage_2.1 : Subsystem  Variant=on
      settings: PortSchema="{\"entries\":[{\"content\":{\"sides\":[{\"content\":{\"connectorIds\":[\"In1\",\"Out2\"]},\"type\":\"ConnectorPlacement.EquallySpacedRectSide\",\"uuid\":\"898fedf9-82f7-4bc2-bf05-880de36b191d\"},{\"content\":{\"connectorIds\":[\"Out1\",\"In2\"],\"side\":\"RIGHT\"},\"type\":\"ConnectorPlacement.EquallySpacedRectSide\",\"uuid\":\"50317b6c-245f-4bd1-a8cd-7a774957ae86\"},{\"content\":{\"side\":\"TOP\"},\"type\":\"ConnectorPlacement.EquallySpacedRectSide\",\"uuid\":\"ff1de2a1-7305-40d8-9e1f-fd0fa1e7d830\"}]},\"type\":\"ConnectorPlacement.EquallySpacedConnector\",\"uuid\":\"6ce82d73-f3da-4f59-9039-464a6ef3e9c5\"}],\"packageUris\":[\"http://schema.mathworks.com/mf0/Connector/R2020b\"],\"version\":\"1.0\"}"
      mask Display: image('images/branco.png');
  Stage_2.2 : Subsystem  Variant=on
      settings: PortSchema="{\"entries\":[{\"content\":{\"sides\":[{\"content\":{\"connectorIds\":[\"In1\",\"Out2\"]},\"type\":\"ConnectorPlacement.EquallySpacedRectSide\",\"uuid\":\"898fedf9-82f7-4bc2-bf05-880de36b191d\"},{\"content\":{\"connectorIds\":[\"Out1\",\"In2\"],\"side\":\"RIGHT\"},\"type\":\"ConnectorPlacement.EquallySpacedRectSide\",\"uuid\":\"50317b6c-245f-4bd1-a8cd-7a774957ae86\"},{\"content\":{\"side\":\"TOP\"},\"type\":\"ConnectorPlacement.EquallySpacedRectSide\",\"uuid\":\"ff1de2a1-7305-40d8-9e1f-fd0fa1e7d830\"}]},\"type\":\"ConnectorPlacement.EquallySpacedConnector\",\"uuid\":\"6ce82d73-f3da-4f59-9039-464a6ef3e9c5\"}],\"packageUris\":[\"http://schema.mathworks.com/mf0/Connector/R2020b\"],\"version\":\"1.0\"}"
      mask Display: image('images/branco.png');
  Stage_3 : Subsystem  Variant=on
      settings: PortSchema="{\"entries\":[{\"content\":{\"sides\":[{\"content\":{\"connectorIds\":[\"In1\",\"Out2\"]},\"type\":\"ConnectorPlacement.EquallySpacedRectSide\",\"uuid\":\"37b17ee8-4b62-4191-976c-22442f171034\"},{\"content\":{\"connectorIds\":[\"Out1\",\"In2\"],\"side\":\"RIGHT\"},\"type\":\"ConnectorPlacement.EquallySpacedRectSide\",\"uuid\":\"4dd88878-371f-49ed-bf90-7ed62e5325b4\"},{\"content\":{\"side\":\"TOP\"},\"type\":\"ConnectorPlacement.EquallySpacedRectSide\",\"uuid\":\"77efb153-e78e-4021-a08b-14751aa491e1\"}]},\"type\":\"ConnectorPlacement.EquallySpacedConnector\",\"uuid\":\"fa13ac12-58ae-4dfa-a455-8cf832864b15\"}],\"packageUris\":[\"http://schema.mathworks.com/mf0/Connector/R2020b\"],\"version\":\"1.0\"}"
      mask Display: image('images/branco.png');
  Switch : Switch  Criteria=u2 > Threshold  SaturateOnIntegerOverflow=off  InputSameDT=off
  M_Diff : Outport
  tag scope: M_GB=global, M_clutch=global, M_stage1=global, i=global, w_engine=global, w_fdbk_Spur11=global, w_fdbk_Spur21=global, w_fdbk_clutch=global, w_fdbk_tra=global
  wires:
  [w_fdbk_Spur21] -> Bus Creator2/7  "w_fdbk_spur21"
  [w_fdbk_Spur11] -> Bus Creator2/6  "w_fdbk_spur11"
  Saturation/1 -> Switch/3
  Divide/1 -> [i]
  Constant2/1 -> Switch/1
  [Take_off] -> Switch/2
  [w_fdbk_diff] -> Saturation/1
  Switch/1 -> Divide/1
  [w_engine] -> Divide/2
  [w_fdbk_diff] -> Bus Creator2/5  "w_fdbk_diff"
  [w_fdbk_axleL] -> Bus Creator2/4  "w_fdbk_axle"
  [w_fdbk_tire] -> Bus Creator2/3  "w_fdbk_tire"
  Bus Creator2/1 -> [w_fdbk_tra]
  [w_clutch] -> Bus Creator2/2  "w_clutch"
  [w_fdbk_S1] -> Bus Creator2/1  "w_fdbk_S1"
  [M_stage1] -> Bus Creator1/1  "M_stage1"
  [M_clutch] -> Bus Creator1/2  "M_clutch"
  Bus Creator1/1 -> [M_GB]
  M_engine/1 -> Stage_1/1(Torque_in)
  Stage_3/1(Torque_out) -> M_Diff/1
  Stage_1/1(Torque_out) -> [M_stage1], Clutch/1(M_in)
  Stage_2.2/1(Torque_out) -> Multiport Switch1/4
  Multiport Switch1/1 -> Stage_3/1(Torque_in)
  Clutch/2(w_in) -> [w_fdbk_clutch], Stage_1/2(Speed_fdbk)
  [w_fdbk_diff] -> Stage_3/2(Speed_fdbk)
  Stage_3/2(Speed_out) -> Stage_2.1/2(Speed_fdbk), Stage_2.2/2(Speed_fdbk)
  Stage_1/2(Speed_out) -> [w_engine]
  [Gear] -> Multiport Switch1/2, Multiport Switch1/1
  Stage_2.1/1(Torque_out) -> Multiport Switch1/3
  Clutch/1(M_clutch) -> Stage_2.1/1(Torque_in), Stage_2.2/1(Torque_in), [M_clutch]
  [Gear] -> Multiport Switch2/1
  Stage_2.1/2(Speed_out) -> [w_fdbk_Spur11], Multiport Switch2/3
  Stage_2.2/2(Speed_out) -> [w_fdbk_Spur21], Multiport Switch2/2, Multiport Switch2/4
  Multiport Switch2/1 -> Clutch/3(w_out)
  [clutch] -> Clutch/2(" ")

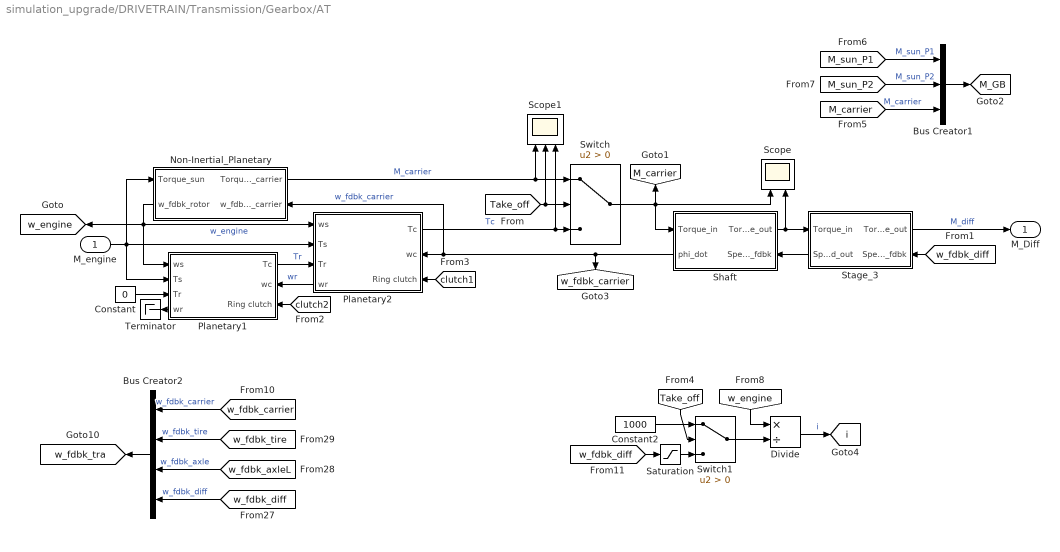
== system simulation_upgrade/DRIVETRAIN/Transmission/Gearbox/AT ==
  M_engine : Inport
  Bus Creator1 : BusCreator  Inputs=3
  Bus Creator2 : BusCreator  Inputs=4
  Constant : Constant  Value=0
  Constant2 : Constant  Value=1000
  Divide : Product  Inputs=*/
  Non-Inertial_Planetary : Subsystem  mask{Zs=Planetary.SunGear.Z, Js=Planetary.SunGear.J, Zr=Planetary.RingGear.Z, Jr=Planetary.RingGear.J, Jc=Planetary.Carrier.J, mp=Planetary.PlanetGear.M, np=Planetary.PlanetGear.N}
      mask prompts: Zs "Sun_Z"; Js "Sun_Inertia"; Zr "Ring_Z"; Jr "Ring_Inertia"; Jc "Carrier_Inertia"; mp "Planet_Mass"; np "Planets_Number"
      settings: PortSchema="{\"entries\":[{\"content\":{\"sides\":[{\"content\":{\"connectorIds\":[\"In1\",\"Out2\"]},\"type\":\"ConnectorPlacement.EquallySpacedRectSide\",\"uuid\":\"c3aadec2-c0b9-48c9-b0c9-f7518b4afca5\"},{\"content\":{\"connectorIds\":[\"Out1\",\"In2\"],\"side\":\"RIGHT\"},\"type\":\"ConnectorPlacement.EquallySpacedRectSide\",\"uuid\":\"e7090851-d8d7-48a0-b377-3350364a2837\"},{\"content\":{\"side\":\"TOP\"},\"type\":\"ConnectorPlacement.EquallySpacedRectSide\",\"uuid\":\"239cd309-0e28-49d0-8c0b-e8c556f33b85\"}]},\"type\":\"ConnectorPlacement.EquallySpacedConnector\",\"uuid\":\"2c7faf18-3f40-4178-83a0-0ad943f67af0\"}],\"packageUris\":[\"http://schema.mathworks.com/mf0/Connector/R2020b\"],\"version\":\"1.0\"}"
  Planetary1 : Subsystem  mask{Zs=Planetary.SunGear.Z, Js=Planetary.SunGear.J, Zr=Planetary.RingGear.Z, Jr=Planetary.RingGear.J, Jc=Planetary.Carrier.J, mp=Planetary.PlanetGear.M, np=Planetary.PlanetGear.N}
      mask prompts: Zs "Sun_Z"; Js "Sun_Inertia"; Zr "Ring_Z"; Jr "Ring_Inertia"; Jc "Carrier_Inertia"; mp "Planet_Mass"; np "Planets_Number"
      settings: PortSchema="{\"entries\":[{\"content\":{\"sides\":[{\"content\":{\"connectorIds\":[\"In1\",\"In2\",\"In3\",\"Out2\"]},\"type\":\"ConnectorPlacement.EquallySpacedRectSide\",\"uuid\":\"c3aadec2-c0b9-48c9-b0c9-f7518b4afca5\"},{\"content\":{\"connectorIds\":[\"Out1\",\"In4\",\"In5\"],\"side\":\"RIGHT\"},\"type\":\"ConnectorPlacement.EquallySpacedRectSide\",\"uuid\":\"e7090851-d8d7-48a0-b377-3350364a2837\"},{\"content\":{\"side\":\"TOP\"},\"type\":\"ConnectorPlacement.EquallySpacedRectSide\",\"uuid\":\"239cd309-0e28-49d0-8c0b-e8c556f33b85\"}]},\"type\":\"ConnectorPlacement.EquallySpacedConnector\",\"uuid\":\"2c7faf18-3f40-4178-83a0-0ad943f67af0\"}],\"packageUris\":[\"http://schema.mathworks.com/mf0/Connector/R2020b\"],\"version\":\"1.0\"}"
  Planetary2 : Subsystem  mask{Zs=Planetary.SunGear.Z, Js=Planetary.SunGear.J, Zr=Planetary.RingGear.Z, Jr=Planetary.RingGear.J, Jc=Planetary.Carrier.J, mp=Planetary.PlanetGear.M, np=Planetary.PlanetGear.N}
      mask prompts: Zs "Sun_Z"; Js "Sun_Inertia"; Zr "Ring_Z"; Jr "Ring_Inertia"; Jc "Carrier_Inertia"; mp "Planet_Mass"; np "Planets_Number"
      settings: PortSchema="{\"entries\":[{\"content\":{\"sides\":[{\"content\":{\"connectorIds\":[\"In1\",\"In2\",\"In3\",\"Out2\"]},\"type\":\"ConnectorPlacement.EquallySpacedRectSide\",\"uuid\":\"c3aadec2-c0b9-48c9-b0c9-f7518b4afca5\"},{\"content\":{\"connectorIds\":[\"Out1\",\"In4\",\"In5\"],\"side\":\"RIGHT\"},\"type\":\"ConnectorPlacement.EquallySpacedRectSide\",\"uuid\":\"e7090851-d8d7-48a0-b377-3350364a2837\"},{\"content\":{\"side\":\"TOP\"},\"type\":\"ConnectorPlacement.EquallySpacedRectSide\",\"uuid\":\"239cd309-0e28-49d0-8c0b-e8c556f33b85\"}]},\"type\":\"ConnectorPlacement.EquallySpacedConnector\",\"uuid\":\"2c7faf18-3f40-4178-83a0-0ad943f67af0\"}],\"packageUris\":[\"http://schema.mathworks.com/mf0/Connector/R2020b\"],\"version\":\"1.0\"}"
  Saturation : Saturate  UpperLimit=100000  LowerLimit=1
  Scope : Scope  NumInputPorts=2
  Scope1 : Scope  NumInputPorts=3
  Shaft : Subsystem  mask{J=Shaft.J}
      mask prompts: J "Inertia_kgm^2"
      settings: PortSchema="{\"entries\":[{\"content\":{\"sides\":[{\"content\":{\"connectorIds\":[\"In1\",\"Out2\"]},\"type\":\"ConnectorPlacement.EquallySpacedRectSide\",\"uuid\":\"898fedf9-82f7-4bc2-bf05-880de36b191d\"},{\"content\":{\"connectorIds\":[\"Out1\",\"In2\"],\"side\":\"RIGHT\"},\"type\":\"ConnectorPlacement.EquallySpacedRectSide\",\"uuid\":\"50317b6c-245f-4bd1-a8cd-7a774957ae86\"},{\"content\":{\"side\":\"TOP\"},\"type\":\"ConnectorPlacement.EquallySpacedRectSide\",\"uuid\":\"ff1de2a1-7305-40d8-9e1f-fd0fa1e7d830\"}]},\"type\":\"ConnectorPlacement.EquallySpacedConnector\",\"uuid\":\"6ce82d73-f3da-4f59-9039-464a6ef3e9c5\"}],\"packageUris\":[\"http://schema.mathworks.com/mf0/Connector/R2020b\"],\"version\":\"1.0\"}"
  Stage_3 : Subsystem  Variant=on
      settings: PortSchema="{\"entries\":[{\"content\":{\"sides\":[{\"content\":{\"connectorIds\":[\"In1\",\"Out2\"]},\"type\":\"ConnectorPlacement.EquallySpacedRectSide\",\"uuid\":\"37b17ee8-4b62-4191-976c-22442f171034\"},{\"content\":{\"connectorIds\":[\"Out1\",\"In2\"],\"side\":\"RIGHT\"},\"type\":\"ConnectorPlacement.EquallySpacedRectSide\",\"uuid\":\"4dd88878-371f-49ed-bf90-7ed62e5325b4\"},{\"content\":{\"side\":\"TOP\"},\"type\":\"ConnectorPlacement.EquallySpacedRectSide\",\"uuid\":\"77efb153-e78e-4021-a08b-14751aa491e1\"}]},\"type\":\"ConnectorPlacement.EquallySpacedConnector\",\"uuid\":\"fa13ac12-58ae-4dfa-a455-8cf832864b15\"}],\"packageUris\":[\"http://schema.mathworks.com/mf0/Connector/R2020b\"],\"version\":\"1.0\"}"
      mask Display: image('images/branco.png');
  Switch : Switch  Criteria=u2 > Threshold  SaturateOnIntegerOverflow=off  InputSameDT=off
  Switch1 : Switch  Criteria=u2 > Threshold  SaturateOnIntegerOverflow=off  InputSameDT=off
  Terminator : Terminator
  M_Diff : Outport
  tag scope: M_GB=global, M_carrier=global, i=global, w_engine=global, w_fdbk_carrier=global, w_fdbk_tra=global
  wires:
  [w_fdbk_diff] -> Stage_3/2(Speed_fdbk)
  Shaft/1(Torque_out) -> Stage_3/1(Torque_in), Scope/2
  Stage_3/1(Torque_out) -> M_Diff/1  "M_diff"
  Stage_3/2(Speed_out) -> Shaft/2(Speed_fdbk)
  Non-Inertial_Planetary/1(Torque_carrier) -> Switch/1, Scope1/1  "M_carrier"
  Shaft/2(phi_dot) -> Planetary2/4(wc), Non-Inertial_Planetary/2(w_fdbk_carrier), [w_fdbk_carrier]  "w_fdbk_carrier"
  Planetary1/1(Tc) -> Planetary2/3(Tr)  "Tr"
  Planetary2/2(wr) -> Planetary1/4(wc)  "wr"
  M_engine/1 -> Non-Inertial_Planetary/1(Torque_sun), Planetary2/2(Ts), Planetary1/2(Ts)
  Constant/1 -> Planetary1/3(Tr)
  [clutch1] -> Planetary2/5(Ring clutch)
  Planetary2/1(Tc) -> Scope1/3, Switch/3  "Tc"
  Planetary1/2(wr) -> Terminator/1
  Switch/1 -> Scope/1, [M_carrier], Shaft/1(Torque_in)
  [Take_off] -> Switch/2, Scope1/2
  [clutch2] -> Planetary1/5(Ring clutch)
  Non-Inertial_Planetary/2(w_fdbk_rotor) -> Planetary2/1(ws), [w_engine], Planetary1/1(ws)  "w_engine"
  [w_fdbk_carrier] -> Bus Creator2/1  "w_fdbk_carrier"
  [w_fdbk_diff] -> Bus Creator2/4  "w_fdbk_diff"
  Bus Creator2/1 -> [w_fdbk_tra]
  [w_fdbk_axleL] -> Bus Creator2/3  "w_fdbk_axle"
  [w_fdbk_tire] -> Bus Creator2/2  "w_fdbk_tire"
  [M_sun_P1] -> Bus Creator1/1  "M_sun_P1"
  [M_sun_P2] -> Bus Creator1/2  "M_sun_P2"
  [M_carrier] -> Bus Creator1/3  "M_carrier"
  Bus Creator1/1 -> [M_GB]
  [w_fdbk_diff] -> Saturation/1
  [Take_off] -> Switch1/2
  Switch1/1 -> Divide/2
  [w_engine] -> Divide/1
  Constant2/1 -> Switch1/1
  Divide/1 -> [i]  "i"
  Saturation/1 -> Switch1/3
